simulink model "CVS_Model"  (R2021a)
(part 6 of 8)

  L- Right Atrium3/RConn1 -- Tricuspid Valve3/LConn1 -- C- Right Atrium3/LConn1
  R- Right Internal Carotid3/LConn1 -- R- Right External Carotid3/LConn1 -- R-Rdial Artery7/LConn1 -- R-Ulnar Artery7/LConn1
  R-R Posterior Tibial Artery3/LConn1 -- R-R Anterior Tibial Artery3/LConn1 -- C- Left Femoral Artery3/LConn1 -- L-Left Femoral Artery3/RConn1
  L-Right Subclavin3/RConn1 -- C-Right Subclavin3/LConn1 -- R- BrachiocephalicArtery3/LConn1 -- L-Right Common Carotid A3/RConn1 -- C-Right Common Carotid A3/LConn1 -- L-Vertebral Artery3/RConn1 -- C-Vertebral Artery3/LConn1
  C-Right Common Iliac3/LConn1 -- R-Right External Iliac3/LConn1 -- L-Right Common Iliac3/RConn1
  R-LIPV3/LConn1 -- R- LSPV3/LConn1 -- L- LPA3/RConn1 -- C- LPA3/LConn1
  C-Ulnar Artery7/LConn1 -- L-Ulnar Artery7/RConn1 -- R- R Brachial3/LConn1 -- L-Radial Artery7/RConn1 -- C-Radial Artery7/LConn1
  C-axilary3/LConn1 -- R- Right Subclavin3/LConn1 -- L-axilary3/RConn1
  L-  Descending Aorta3/RConn1 -- C- Descending Aorta3/LConn1 -- R-  Abdominal Aorta3/LConn1
  L- Inferior Vena Cava3/RConn1 -- C- Inferior Vena Cava3/LConn1 -- R- Right Atrium3/LConn1 -- L- Superior Vena Cava3/RConn1 -- C- Superoir Vena Cava3/LConn1
  Solver Configuration3/RConn1 -- R-Right Pulmonary Artery3/LConn1 -- C- main Pulmonary Artery3/LConn1 -- L- main Pulmonary Artery3/RConn1 -- R- left Pulmonary Artery3/LConn1
  C-BrachiocephalicArtery3/LConn1 -- L-BrachiocephalicArtery3/RConn1 -- L3/LConn1
  Mitral Valve3/RConn1 -- DC Voltage Source7/LConn1 -- Resistor15/LConn1
  L-3/RConn1 -- R- Left Vertebral3/LConn1 -- R- Left Subcalvin 4/LConn1
  R- Axillary3/LConn1 -- L-Left Subcalvin4/RConn1 -- C-Left Subcalvin4/LConn1
  L-Right External Iliac3/RConn1 -- R-Right Femoral Artery3/LConn1 -- C-Right External Iliac3/LConn1
  L R Brachial3/RConn1 -- R- axilary3/LConn1 -- C- R Brachial3/LConn1
  C- Left Atrium3/LConn1 -- Mitral Valve3/LConn1 -- L- Left Atrium3/RConn1
  R- Right Ventricle3/LConn1 -- DC Voltage Source8/LConn1 -- Tricuspid Valve3/RConn1
  C- Brachial3/RConn1 -- R- visco  Brachial3/LConn1
  L- RSPV3/LConn1 -- R- RSPV3/RConn1
  PS-Simulink Converter19/LConn1 -- Voltage Sensor19/RConn1
  R- Right External Carotid3/RConn1 -- L-Right External Carotid3/LConn1
  Electrical Reference203/LConn1 -- C- LSPV3/RConn1
  R-R Anterior Tibial Artery3/RConn1 -- L- R Anterior Tibial Artery3/LConn1
  R- Right Common Carotid A 3/RConn1 -- L-Right Common Carotid A3/LConn1
  R-Ulnar Artery7/RConn1 -- L-Ulnar Artery7/LConn1
  R- Viscoelastic3/RConn1 -- Electrical Reference209/LConn1
  Electrical Reference226/LConn1 -- R-Visco Right Gastric3/RConn1
  R- visco Axilary3/RConn1 -- Electrical Reference223/LConn1
  L-LSPV3/LConn1 -- R- LSPV3/RConn1
  C- main Pulmonary Artery3/RConn1 -- R- Viscoelastic3/LConn1
  Electrical Reference212/LConn1 -- Resistor19/RConn1
  C- Posterior Tibial Artery3/RConn1 -- R-Visco PT3/LConn1
  R-Visco RCI3/LConn1 -- C-Right Common Iliac3/RConn1
  Voltage Sensor18/RConn1 -- PS-Simulink Converter18/LConn1
  R- Ulnar Artery7/RConn1 -- Electrical Reference193/LConn1
  R-LIPV3/RConn1 -- L -LIPV3/LConn1
  Capacitor9/RConn1 -- Electrical Reference205/LConn1
  C-Ulnar Artery6/RConn1 -- R- Ulnar Artery6/LConn1
  C- Abdominal Aorta 4/RConn1 -- R-Viscoelastic AB4/LConn1
  C- Right Atrium3/RConn1 -- Electrical Reference214/LConn1
  Voltage Sensor18/RConn2 -- Electrical Reference216/LConn1
  C-BrachiocephalicArtery3/RConn1 -- R- visco BrachiocephalicArtery3/LConn1
  Electrical Reference232/LConn1 -- R-Visco SM3/RConn1
  R- visco Left Vertebral3/RConn1 -- Electrical Reference200/LConn1
  C-Ulnar Artery7/RConn1 -- R- Ulnar Artery7/LConn1
  R-RIPV3/RConn1 -- L- RIPV3/LConn1
  R- visco  Brachial3/RConn1 -- Electrical Reference224/LConn1
  R- Superior Vena Cava9/LConn1 -- R- Superior Vena Cava10/RConn1
  R-Visco PT3/RConn1 -- Electrical Reference242/LConn1
  R-Visco SM3/LConn1 -- C- Superior Mesentric3/RConn1
  Pulmonary Valve3/RConn1 -- R- main Pulmonary Artery3/LConn1
  R- Vertebral Artery3/RConn1 -- L-Vertebral Artery3/LConn1
  L- main Pulmonary Artery3/LConn1 -- R- main Pulmonary Artery3/RConn1
  R- Splentic3/RConn1 -- L-Splentic3/LConn1
  R-Visco IM3/RConn1 -- Electrical Reference233/LConn1
  Controlled Voltage Source8/LConn1 -- DC Voltage Source8/RConn1
  R-Rdial Artery7/RConn1 -- L-Radial Artery7/LConn1
  C-  L Anterior Tibial Artery3/RConn1 -- R- L Visco AT3/LConn1
  L-  Abdominal Aorta 4/LConn1 -- R-  Abdominal Aorta3/RConn1
  R-Visco LFA3/RConn1 -- Electrical Reference238/LConn1
  R-Visco LCI3/LConn1 -- C- Left Common Iliac3/RConn1
  R- Brachial3/RConn1 -- L- Brachial3/LConn1
  R-L Anterior Tibial Artery3/RConn1 -- L- L Anterior Tibial Artery3/LConn1
  R- visco VA3/RConn1 -- Electrical Reference192/LConn1
  C-Radial Artery6/RConn1 -- R- Radial Artery6/LConn1
  L R Brachial3/LConn1 -- R- R Brachial3/RConn1
  Simulink-PS Converter8/RConn1 -- Controlled Voltage Source8/RConn1
  R- Hepatic Artery3/RConn1 -- L-  Hepatic Artery3/LConn1
  L- RPA3/LConn1 -- R-Right Pulmonary Artery3/RConn1
  C-Right Subclavin3/RConn1 -- R- visco RS3/LConn1
  L-Inferior Mesentric3/LConn1 -- R- Inferior Mesentric3/RConn1
  R-  R Brachial3/RConn1 -- Electrical Reference187/LConn1
  C-Right Common Carotid A3/RConn1 -- R- visco RCCA3/LConn1
  C- Anterior Tibial Artery3/RConn1 -- R-Visco AT3/LConn1
  Electrical Reference219/LConn1 -- R-Viscoelastic DA3/RConn1
  R-Visco RCI3/RConn1 -- Electrical Reference235/LConn1
  C- R Brachial3/RConn1 -- R-  R Brachial3/LConn1
  R- Ulnar Artery6/RConn1 -- Electrical Reference201/LConn1
  R- visco BrachiocephalicArtery3/RConn1 -- Electrical Reference190/LConn1
  R-Visco LFA3/LConn1 -- C- Left Femoral Artery3/RConn1
  L-L Posterior Tibial Artery3/LConn1 -- R-L Posterior Tibial Artery3/RConn1
  C-Right External Carotid3/RConn1 -- R- visco REC3/LConn1
  R- visco RS3/RConn1 -- Electrical Reference194/LConn1
  R-Visco Left Gastric3/RConn1 -- Electrical Reference227/LConn1
  R-Left Femoral Artery3/RConn1 -- L-Left Femoral Artery3/LConn1
  C-Radial Artery7/RConn1 -- R- Radial Artery7/LConn1
  R-Left Gastric Artery3/RConn1 -- L-Left Gastric Artery3/LConn1
  Electrical Reference206/LConn1 -- Controlled Voltage Source7/RConn2
  R- Superior Mesentric3/RConn1 -- L-Superior Mesentric3/LConn1
  L- Right Ventricle3/LConn1 -- R- Right Ventricle3/RConn1
  Resistor16/RConn1 -- Inductor11/LConn1
  L- Inferior Vena Cava3/LConn1 -- R- Inferior Vena Cava3/RConn1
  Electrical Reference186/LConn1 -- R- Radial Artery7/RConn1
  L-  Descending Aorta3/LConn1 -- R- Descending Aorta3/RConn1
  Inductor9/LConn1 -- Resistor15/RConn1
  L-Left Common Iliac3/LConn1 -- R-Left Common Iliac3/RConn1
  Electrical Reference208/LConn1 -- C- Right Ventricle3/RConn1
  R- Left Vertebral3/RConn1 -- L-Left Vertebral3/LConn1
  L-axilary3/LConn1 -- R- axilary3/RConn1
  R- Inferior Vena Cava3/LConn1 -- R- Superior Vena Cava11/LConn1
  Simulink-PS Converter7/RConn1 -- Controlled Voltage Source7/RConn1
  Resistor19/LConn1 -- Capacitor10/RConn1
  Resistor17/RConn1 -- Inductor10/LConn1
  R-Visco LR3/RConn1 -- Electrical Reference231/LConn1
  Electrical Reference188/LConn1 -- Resistor18/RConn1
  R-Rdial Artery6/RConn1 -- L-Radial Artery6/LConn1
  R-Visco LEI3/RConn1 -- Electrical Reference236/LConn1
  C-Vertebral Artery3/RConn1 -- R- visco VA3/LConn1
  C-Right Internal Carotid3/RConn1 -- R- visco RIC3/LConn1
  R-Visco Right Gastric3/LConn1 -- C- Right Gastric Artery3/RConn1
  R-Visco RFA3/LConn1 -- C-Right Femoral Artery3/RConn1
  C- RIPV3/RConn1 -- Electrical Reference202/LConn1
  R-Visco LR3/LConn1 -- C-  Left Renal Artery3/RConn1
  Electrical Reference220/LConn1 -- C- Inferior Vena Cava3/RConn1
  C- Left Atrium3/RConn1 -- Electrical Reference239/LConn1
  R- Left Subcalvin 4/RConn1 -- L-Left Subcalvin4/LConn1
  L-Right External Iliac3/LConn1 -- R-Right External Iliac3/RConn1
  R- visco axilary3/RConn1 -- Electrical Reference185/LConn1
  R-Left External Iliac3/RConn1 -- L-Left External Iliac3/LConn1
  Electrical Reference218/LConn1 -- R-Viscoelastic AB4/RConn1
  C- L Posterior Tibial Artery3/RConn1 -- R-L Visco PT3/LConn1
  R- Right Gastric Artery3/RConn1 -- L- Right Gastric Artery3/LConn1
  R-Visco REI3/RConn1 -- Electrical Reference237/LConn1
  C- Descending Aorta3/RConn1 -- R-Viscoelastic DA3/LConn1
  R- visco RCCA3/RConn1 -- Electrical Reference191/LConn1
  R- BrachiocephalicArtery3/RConn1 -- L-BrachiocephalicArtery3/LConn1
  Electrical Reference221/LConn1 -- R- visco Left Subcalvin4/RConn1
  C-Left Subcalvin4/RConn1 -- R- visco Left Subcalvin4/LConn1
  R-Visco Hepatic 3/LConn1 -- C- Hepatic Artery3/RConn1
  R- Right Atrium3/RConn1 -- L- Right Atrium3/LConn1
  R-Visco LCI3/RConn1 -- Electrical Reference234/LConn1
  R-Visco LEI3/LConn1 -- C- Left External Iliac3/RConn1
  C- Inferior Mesentric3/RConn1 -- R-Visco IM3/LConn1
  R-Visco Splentic3/RConn1 -- Electrical Reference229/LConn1
  L-R Posterior Tibial Artery3/LConn1 -- R-R Posterior Tibial Artery3/RConn1
  C- LPA3/RConn1 -- R- LPA3/LConn1
  L-Right Femoral Artery3/LConn1 -- R-Right Femoral Artery3/RConn1
  R- Right Internal Carotid3/RConn1 -- L-Right Internal Carotid3/LConn1
  R-Visco Splentic3/LConn1 -- C- Splentic3/RConn1
  R- Superior Vena Cava9/RConn1 -- L- Superior Vena Cava3/LConn1
  R-Visco RFA3/RConn1 -- Electrical Reference240/LConn1
  R- L Visco AT3/RConn1 -- Electrical Reference243/LConn1
  L- LPA3/LConn1 -- R- left Pulmonary Artery3/RConn1
  C- Superoir Vena Cava3/RConn1 -- Electrical Reference215/LConn1
  R-Visco RR3/LConn1 -- C- Right Renal Artery3/RConn1
  R-Visco Left Gastric3/LConn1 -- C- Left Gastric Artery3/RConn1
  C-Left Vertebral3/RConn1 -- R- visco Left Vertebral3/LConn1
  C- RPA3/RConn1 -- R-R Viscielastic3/LConn1
  C-Axilary3/RConn1 -- R- visco Axilary3/LConn1
  R- visco REC3/RConn1 -- Electrical Reference196/LConn1
  R- Left Atrium3/RConn1 -- L- Left Atrium3/LConn1
  R-Visco AT3/RConn1 -- Electrical Reference241/LConn1
  Electrical Reference210/LConn1 -- R- Radial Artery6/RConn1
  R-Visco REI3/LConn1 -- C-Right External Iliac3/RConn1
  C- RSPV3/RConn1 -- Electrical Reference199/LConn1
  Electrical Reference225/LConn1 -- R-Visco Hepatic 3/RConn1
  R- visco RIC3/RConn1 -- Electrical Reference195/LConn1
  R- Axillary3/RConn1 -- L-Axillary3/LConn1
  R- Right Renal Artery3/RConn1 -- L-Right Renal Artery3/LConn1
  R- LPA3/RConn1 -- Electrical Reference189/LConn1
  R- Left Renal Artery3/RConn1 -- L- Left Renal Artery3/LConn1
  Voltage Sensor19/RConn2 -- Electrical Reference213/LConn1
  Resistor18/LConn1 -- Capacitor11/RConn1
  L-Right Common Iliac3/LConn1 -- R-Right Common Iliac3/RConn1
  R- Right Subclavin3/RConn1 -- L-Right Subclavin3/LConn1
  R-R Viscielastic3/RConn1 -- Electrical Reference207/LConn1
  Electrical Reference204/LConn1 -- C-LIPV3/RConn1
  R-Visco RR3/RConn1 -- Electrical Reference230/LConn1
  R-Ulnar Artery6/RConn1 -- L-Ulnar Artery6/LConn1
  DC Voltage Source7/RConn1 -- Controlled Voltage Source7/LConn1
  C-axilary3/RConn1 -- R- visco axilary3/LConn1
  R-L Visco PT3/RConn1 -- Electrical Reference183/LConn1
  Diode3/RConn1 -- Resistor12/LConn1
  R-Rdial Artery8/LConn1 -- R-Ulnar Artery8/LConn1 -- C- Brachial4/LConn1 -- L- Brachial4/RConn1
  L-Ulnar Artery9/RConn1 -- C-Ulnar Artery9/LConn1 -- R- R Brachial4/LConn1 -- L-Radial Artery9/RConn1 -- C-Radial Artery9/LConn1
  C-Radial Artery8/LConn1 -- C-Ulnar Artery8/LConn1 -- L-Ulnar Artery8/RConn1 -- R- Vertebral Artery4/LConn1 -- R- Superior Vena Cava13/LConn1 -- C-Left Vertebral4/LConn1 -- L-Left Vertebral4/RConn1 -- Voltage Sensor23/LConn1 -- L-Radial Artery8/RConn1
  L-Left External Iliac4/RConn1 -- C- Left External Iliac4/LConn1 -- R-Left Femoral Artery4/LConn1
  C-Right Common Carotid A4/LConn1 -- L-Right Common Carotid A4/RConn1 -- R- BrachiocephalicArtery4/LConn1 -- C-Vertebral Artery4/LConn1 -- L-Vertebral Artery4/RConn1 -- C-Right Subclavin4/LConn1 -- L-Right Subclavin4/RConn1
  L4/LConn1 -- C-BrachiocephalicArtery4/LConn1 -- L-BrachiocephalicArtery4/RConn1
  Capacitor13/LConn1 -- L4/RConn1 -- Resistor21/LConn1 -- Inductor13/RConn1 -- Voltage Sensor22/LConn1
  Resistor20/LConn1 -- Mitral Valve5/RConn1 -- DC Voltage Source9/LConn1
  C-Left Subcalvin5/LConn1 -- R- Axillary4/LConn1 -- L-Left Subcalvin5/RConn1
  C-Right Femoral Artery4/LConn1 -- L-Right Femoral Artery4/RConn1 -- R-L Posterior Tibial Artery4/LConn1 -- R-L Anterior Tibial Artery4/LConn1
  R-R Anterior Tibial Artery4/LConn1 -- R-R Posterior Tibial Artery4/LConn1 -- C- Left Femoral Artery4/LConn1 -- L-Left Femoral Artery4/RConn1
  R- Superior Mesentric4/LConn1 -- R- Right Renal Artery4/LConn1 -- R- Left Renal Artery4/LConn1 -- R- Inferior Mesentric4/LConn1 -- C- L Posterior Tibial Artery4/LConn1 -- L-L Posterior Tibial Artery4/RConn1 -- C-  L Anterior Tibial Artery4/LConn1 -- L- L Anterior Tibial Artery4/RConn1 -- L- R Anterior Tibial Artery4/RConn1 -- C- Anterior Tibial Artery4/LConn1 -- C- Posterior Tibial Artery4/LConn1 -- L-R Posterior Tibial Artery4/RConn1 -- R- Superior Vena Cava14/RConn1 -- R- Right Gastric Artery4/LConn1 -- R- Hepatic Artery4/LConn1 -- R-Left Gastric Artery4/LConn1 -- R- Splentic4/LConn1
  R- Left Subcalvin 5/LConn1 -- L-4/RConn1 -- R- Left Vertebral4/LConn1
  C- Right Ventricle4/LConn1 -- L- Right Ventricle4/RConn1 -- Pulmonary Valve4/LConn1
  C- Right Atrium4/LConn1 -- L- Right Atrium4/RConn1 -- Tricuspid Valve4/LConn1
  L- Left Atrium4/RConn1 -- C- Left Atrium4/LConn1 -- Mitral Valve5/LConn1
  C- LPA4/LConn1 -- L- LPA4/RConn1 -- R-LIPV4/LConn1 -- R- LSPV4/LConn1
  Inductor14/RConn1 -- Capacitor14/LConn1 -- R- Descending Aorta4/LConn1 -- L-4/LConn1
  R- left Pulmonary Artery4/LConn1 -- C- main Pulmonary Artery4/LConn1 -- L- main Pulmonary Artery4/RConn1 -- Solver Configuration4/RConn1 -- R-Right Pulmonary Artery4/LConn1
  R-Ulnar Artery9/LConn1 -- R-Rdial Artery9/LConn1 -- R- Right Internal Carotid4/LConn1 -- R- Right External Carotid4/LConn1
  C- Superoir Vena Cava4/LConn1 -- L- Superior Vena Cava4/RConn1 -- R- Right Atrium4/LConn1 -- L- Inferior Vena Cava4/RConn1 -- C- Inferior Vena Cava4/LConn1
  C- R Brachial4/LConn1 -- L R Brachial4/RConn1 -- R- axilary4/LConn1
  L-Right Common Iliac4/RConn1 -- C-Right Common Iliac4/LConn1 -- R-Right External Iliac4/LConn1
  L-axilary4/RConn1 -- C-axilary4/LConn1 -- R- Right Subclavin4/LConn1
  C- RSPV4/LConn1 -- L- RSPV4/RConn1 -- C- RIPV4/LConn1 -- L- RIPV4/RConn1 -- R- Left Atrium4/LConn1 -- L -LIPV4/RConn1 -- C-LIPV4/LConn1 -- L-LSPV4/RConn1 -- C- LSPV4/LConn1
  Tricuspid Valve4/RConn1 -- R- Right Ventricle4/LConn1 -- DC Voltage Source10/LConn1
  R- RSPV4/LConn1 -- L- RPA4/RConn1 -- C- RPA4/LConn1 -- R-RIPV4/LConn1
  C-Right External Carotid4/LConn1 -- R- Right Common Carotid A 4/LConn1 -- L-Right Internal Carotid4/RConn1 -- C-Right Internal Carotid4/LConn1 -- L-Right External Carotid4/RConn1
  C- Abdominal Aorta 5/LConn1 -- L-  Abdominal Aorta 5/RConn1 -- C- Superior Mesentric4/LConn1 -- L-Superior Mesentric4/RConn1 -- C-  Left Renal Artery4/LConn1 -- L- Left Renal Artery4/RConn1 -- C- Right Renal Artery4/LConn1 -- L-Right Renal Artery4/RConn1 -- C- Inferior Mesentric4/LConn1 -- L-Inferior Mesentric4/RConn1 -- R-Left Common Iliac4/LConn1 -- R-Right Common Iliac4/LConn1 -- C- Hepatic Artery4/LConn1 -- L-  Hepatic Artery4/RConn1 -- L- Right Gastric Artery4/RConn1 -- C- Right Gastric Artery4/LConn1 -- C- Splentic4/LConn1 -- L-Splentic4/RConn1 -- L-Left Gastric Artery4/RConn1 -- C- Left Gastric Artery4/LConn1
  L-Left Common Iliac4/RConn1 -- C- Left Common Iliac4/LConn1 -- R-Left External Iliac4/LConn1
  R-  Abdominal Aorta4/LConn1 -- L-  Descending Aorta4/RConn1 -- C- Descending Aorta4/LConn1
  C-Axilary4/LConn1 -- R- Brachial4/LConn1 -- L-Axillary4/RConn1
  C-Right External Iliac4/LConn1 -- L-Right External Iliac4/RConn1 -- R-Right Femoral Artery4/LConn1
  Capacitor12/LConn1 -- Diode/LConn1 -- Inductor12/RConn1
  Diode/RConn1 -- Resistor22/LConn1
  C- RIPV4/RConn1 -- Electrical Reference293/LConn1
  Electrical Reference136/LConn1 -- C- Right Ventricle4/RConn1
  C-  L Anterior Tibial Artery4/RConn1 -- R- L Visco AT4/LConn1
  C- Descending Aorta4/RConn1 -- R-Viscoelastic DA4/LConn1
  L- RSPV4/LConn1 -- R- RSPV4/RConn1
  R- Ulnar Artery8/RConn1 -- Electrical Reference292/LConn1
  C- RPA4/RConn1 -- R-R Viscielastic4/LConn1
  R- BrachiocephalicArtery4/RConn1 -- L-BrachiocephalicArtery4/LConn1
  R- Left Renal Artery4/RConn1 -- L- Left Renal Artery4/LConn1
  Resistor23/LConn1 -- Capacitor14/RConn1
  C-Ulnar Artery8/RConn1 -- R- Ulnar Artery8/LConn1
  Electrical Reference251/LConn1 -- R- visco Left Subcalvin5/RConn1
  R- Right Gastric Artery4/RConn1 -- L- Right Gastric Artery4/LConn1
  R- LPA4/RConn1 -- Electrical Reference280/LConn1
  C-axilary4/RConn1 -- R- visco axilary4/LConn1
  Inductor12/LConn1 -- Resistor20/RConn1
  R- visco VA4/RConn1 -- Electrical Reference283/LConn1
  L R Brachial4/LConn1 -- R- R Brachial4/RConn1
  R- visco Axilary4/RConn1 -- Electrical Reference253/LConn1
  R- visco BrachiocephalicArtery4/RConn1 -- Electrical Reference281/LConn1
  R- visco  Brachial4/RConn1 -- Electrical Reference254/LConn1
  R-Visco LEI4/RConn1 -- Electrical Reference266/LConn1
  C-Right Internal Carotid4/RConn1 -- R- visco RIC4/LConn1
  Electrical Reference255/LConn1 -- R-Visco Hepatic 4/RConn1
  R-Visco RCI4/RConn1 -- Electrical Reference265/LConn1
  R-L Visco PT4/RConn1 -- Electrical Reference274/LConn1
  Electrical Reference294/LConn1 -- C- LSPV4/RConn1
  L-LSPV4/LConn1 -- R- LSPV4/RConn1
  R-Visco LR4/RConn1 -- Electrical Reference261/LConn1
  C-Radial Artery8/RConn1 -- R- Radial Artery8/LConn1
  C- Right Atrium4/RConn1 -- Electrical Reference244/LConn1
  R-L Anterior Tibial Artery4/RConn1 -- L- L Anterior Tibial Artery4/LConn1
  L- LPA4/LConn1 -- R- left Pulmonary Artery4/RConn1
  R- Right Common Carotid A 4/RConn1 -- L-Right Common Carotid A4/LConn1
  C- Superoir Vena Cava4/RConn1 -- Electrical Reference245/LConn1
  R-Visco REI4/RConn1 -- Electrical Reference267/LConn1
  R-Rdial Artery8/RConn1 -- L-Radial Artery8/LConn1
  L- main Pulmonary Artery4/LConn1 -- R- main Pulmonary Artery4/RConn1
  C-Ulnar Artery9/RConn1 -- R- Ulnar Artery9/LConn1
  C-Vertebral Artery4/RConn1 -- R- visco VA4/LConn1
  R-Visco RFA4/RConn1 -- Electrical Reference270/LConn1
  R- visco RIC4/RConn1 -- Electrical Reference286/LConn1
  R-Visco LEI4/LConn1 -- C- Left External Iliac4/RConn1
  Electrical Reference249/LConn1 -- R-Viscoelastic DA4/RConn1
  R- Right Internal Carotid4/RConn1 -- L-Right Internal Carotid4/LConn1
  R- Superior Mesentric4/RConn1 -- L-Superior Mesentric4/LConn1
  L-Left Common Iliac4/LConn1 -- R-Left Common Iliac4/RConn1
  R-Left External Iliac4/RConn1 -- L-Left External Iliac4/LConn1
  L-Right External Iliac4/LConn1 -- R-Right External Iliac4/RConn1
  R- Hepatic Artery4/RConn1 -- L-  Hepatic Artery4/LConn1
  C- Posterior Tibial Artery4/RConn1 -- R-Visco PT4/LConn1
  C-Right Common Carotid A4/RConn1 -- R- visco RCCA4/LConn1
  L-Right Femoral Artery4/LConn1 -- R-Right Femoral Artery4/RConn1
  L- RPA4/LConn1 -- R-Right Pulmonary Artery4/RConn1
  Simulink-PS Converter10/RConn1 -- Controlled Voltage Source10/RConn1
  Resistor24/LConn1 -- Capacitor13/RConn1
  C- R Brachial4/RConn1 -- R-  R Brachial4/LConn1
  R- visco Left Vertebral4/RConn1 -- Electrical Reference291/LConn1
  R-Visco Splentic4/RConn1 -- Electrical Reference259/LConn1
  R- L Visco AT4/RConn1 -- Electrical Reference273/LConn1
  Electrical Reference279/LConn1 -- Resistor23/RConn1
  R-Visco LCI4/LConn1 -- C- Left Common Iliac4/RConn1
  C- LPA4/RConn1 -- R- LPA4/LConn1
  R- visco REC4/RConn1 -- Electrical Reference287/LConn1
  R- Ulnar Artery9/RConn1 -- Electrical Reference284/LConn1
  Electrical Reference198/LConn1 -- Resistor24/RConn1
  L- Right Ventricle4/LConn1 -- R- Right Ventricle4/RConn1
  C-Right External Carotid4/RConn1 -- R- visco REC4/LConn1
  C-Right Subclavin4/RConn1 -- R- visco RS4/LConn1
  Electrical Reference114/LConn1 -- Controlled Voltage Source9/RConn2
  R-Ulnar Artery8/RConn1 -- L-Ulnar Artery8/LConn1
  C-Axilary4/RConn1 -- R- visco Axilary4/LConn1
  L-Right Common Iliac4/LConn1 -- R-Right Common Iliac4/RConn1
  L-  Descending Aorta4/LConn1 -- R- Descending Aorta4/RConn1
  R-Visco Right Gastric4/LConn1 -- C- Right Gastric Artery4/RConn1
  C- L Posterior Tibial Artery4/RConn1 -- R-L Visco PT4/LConn1
  Pulmonary Valve4/RConn1 -- R- main Pulmonary Artery4/LConn1
  R- Right Renal Artery4/RConn1 -- L-Right Renal Artery4/LConn1
  R-Visco LFA4/LConn1 -- C- Left Femoral Artery4/RConn1
  R-Visco RR4/RConn1 -- Electrical Reference260/LConn1
  R- visco RS4/RConn1 -- Electrical Reference285/LConn1
  R- Vertebral Artery4/RConn1 -- L-Vertebral Artery4/LConn1
  Electrical Reference248/LConn1 -- R-Viscoelastic AB5/RConn1
  C-Radial Artery9/RConn1 -- R- Radial Artery9/LConn1
  R- Inferior Vena Cava4/LConn1 -- R- Superior Vena Cava14/LConn1
  R-Rdial Artery9/RConn1 -- L-Radial Artery9/LConn1
  R- Left Vertebral4/RConn1 -- L-Left Vertebral4/LConn1
  R- Axillary4/RConn1 -- L-Axillary4/LConn1
  C-Left Vertebral4/RConn1 -- R- visco Left Vertebral4/LConn1
  Electrical Reference295/LConn1 -- C-LIPV4/RConn1
  DC Voltage Source9/RConn1 -- Controlled Voltage Source9/LConn1
  Electrical Reference161/LConn1 -- R- Radial Artery8/RConn1
  Capacitor12/RConn1 -- Electrical Reference78/LConn1
  R-Visco SM4/LConn1 -- C- Superior Mesentric4/RConn1
  C- Anterior Tibial Artery4/RConn1 -- R-Visco AT4/LConn1
  L-axilary4/LConn1 -- R- axilary4/RConn1
  Electrical Reference262/LConn1 -- R-Visco SM4/RConn1
  R- visco axilary4/RConn1 -- Electrical Reference276/LConn1
  R-LIPV4/RConn1 -- L -LIPV4/LConn1
  R-  R Brachial4/RConn1 -- Electrical Reference278/LConn1
  Resistor22/RConn1 -- Inductor13/LConn1
  R- Right External Carotid4/RConn1 -- L-Right External Carotid4/LConn1
  L-R Posterior Tibial Artery4/LConn1 -- R-R Posterior Tibial Artery4/RConn1
  C- Left Atrium4/RConn1 -- Electrical Reference269/LConn1
  C- main Pulmonary Artery4/RConn1 -- R- Viscoelastic4/LConn1
  R-Visco PT4/RConn1 -- Electrical Reference272/LConn1
  R-Visco Left Gastric4/LConn1 -- C- Left Gastric Artery4/RConn1
  R-RIPV4/RConn1 -- L- RIPV4/LConn1
  L-  Abdominal Aorta 5/LConn1 -- R-  Abdominal Aorta4/RConn1
  C-BrachiocephalicArtery4/RConn1 -- R- visco BrachiocephalicArtery4/LConn1
  C- RSPV4/RConn1 -- Electrical Reference290/LConn1
  C- Brachial4/RConn1 -- R- visco  Brachial4/LConn1
  R-Visco REI4/LConn1 -- C-Right External Iliac4/RConn1
  R-Visco Hepatic 4/LConn1 -- C- Hepatic Artery4/RConn1
  L- Inferior Vena Cava4/LConn1 -- R- Inferior Vena Cava4/RConn1
  R- Splentic4/RConn1 -- L-Splentic4/LConn1
  PS-Simulink Converter23/LConn1 -- Voltage Sensor23/RConn1
  Voltage Sensor23/RConn2 -- Electrical Reference222/LConn1
  Resistor21/RConn1 -- Inductor14/LConn1
  Simulink-PS Converter9/RConn1 -- Controlled Voltage Source9/RConn1
  R- Left Atrium4/RConn1 -- L- Left Atrium4/LConn1
  R- Superior Vena Cava12/RConn1 -- L- Superior Vena Cava4/LConn1
  L-L Posterior Tibial Artery4/LConn1 -- R-L Posterior Tibial Artery4/RConn1
  R- Right Subclavin4/RConn1 -- L-Right Subclavin4/LConn1
  R-Ulnar Artery9/RConn1 -- L-Ulnar Artery9/LConn1
  R-Visco RFA4/LConn1 -- C-Right Femoral Artery4/RConn1
  R- visco RCCA4/RConn1 -- Electrical Reference282/LConn1
  Voltage Sensor22/RConn1 -- PS-Simulink Converter22/LConn1
  R-Left Gastric Artery4/RConn1 -- L-Left Gastric Artery4/LConn1
  R-Visco Left Gastric4/RConn1 -- Electrical Reference257/LConn1
  R-Left Femoral Artery4/RConn1 -- L-Left Femoral Artery4/LConn1
  Electrical Reference277/LConn1 -- R- Radial Artery9/RConn1
  C-Left Subcalvin5/RConn1 -- R- visco Left Subcalvin5/LConn1
  R-Visco RCI4/LConn1 -- C-Right Common Iliac4/RConn1
  Voltage Sensor22/RConn2 -- Electrical Reference246/LConn1
  C- Inferior Mesentric4/RConn1 -- R-Visco IM4/LConn1
  R-Visco AT4/RConn1 -- Electrical Reference271/LConn1
  Electrical Reference250/LConn1 -- C- Inferior Vena Cava4/RConn1
  R- Right Atrium4/RConn1 -- L- Right Atrium4/LConn1
  R- Superior Vena Cava12/LConn1 -- R- Superior Vena Cava13/RConn1
  R-Visco LFA4/RConn1 -- Electrical Reference268/LConn1
  Electrical Reference256/LConn1 -- R-Visco Right Gastric4/RConn1
  R-R Anterior Tibial Artery4/RConn1 -- L- R Anterior Tibial Artery4/LConn1
  R-Visco LCI4/RConn1 -- Electrical Reference264/LConn1
  R- Brachial4/RConn1 -- L- Brachial4/LConn1
  Controlled Voltage Source10/LConn1 -- DC Voltage Source10/RConn1
  L-Inferior Mesentric4/LConn1 -- R- Inferior Mesentric4/RConn1
  C- Abdominal Aorta 5/RConn1 -- R-Viscoelastic AB5/LConn1
  R-R Viscielastic4/RConn1 -- Electrical Reference115/LConn1
  R-Visco IM4/RConn1 -- Electrical Reference263/LConn1
  R-Visco RR4/LConn1 -- C- Right Renal Artery4/RConn1
  R- Viscoelastic4/RConn1 -- Electrical Reference137/LConn1
  R-Visco LR4/LConn1 -- C-  Left Renal Artery4/RConn1
  R-Visco Splentic4/LConn1 -- C- Splentic4/RConn1
  R- Left Subcalvin 5/RConn1 -- L-Left Subcalvin5/LConn1
  Controlled Voltage Source10/RConn2 -- Electrical Reference258/LConn1
  Controlled Voltage Source4/RConn2 -- Electrical Reference84/LConn1
  Controlled Voltage Source6/RConn2 -- Electrical Reference167/LConn1
  Controlled Voltage Source8/RConn2 -- Electrical Reference228/LConn1
  Diode2/RConn1 -- Resistor17/LConn1
